simulink library "syl_grc"  (R2024a)
settings: Solver=VariableStepAuto  StartTime=0.0  StopTime=10.0  RelTol=1e-3
undefined symbols (not defined in the file or in its folder): ASYL_TrqMax_X_V, ASYL_TrqMax_Y_rpm, ASYL_TrqMin_X_V, ASYL_TrqMin_Y_rpm, KSYL_frqSwitchMax_Hz, KSYL_nTMSpdMax_RPM, KSYL_nTMSpdMin_RPM, MINUSONE_FLOAT, MSYL_TrqMax_Z_Nm, MSYL_TrqMin_Z_Nm
libraries: simulink x3
settings Model: Creator=FVT24180  LastModifiedBy=FVT22063

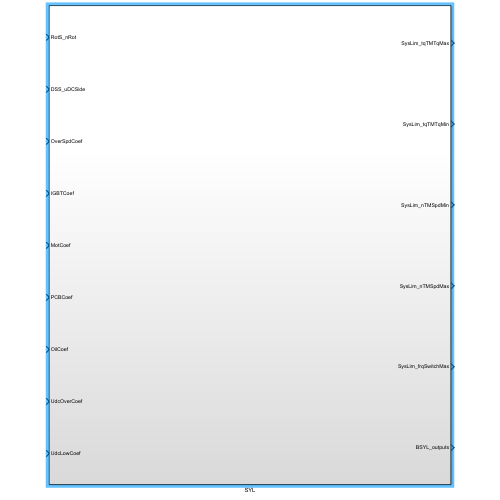
[thumbnail: Simulink's stored preview of the top-level diagram]
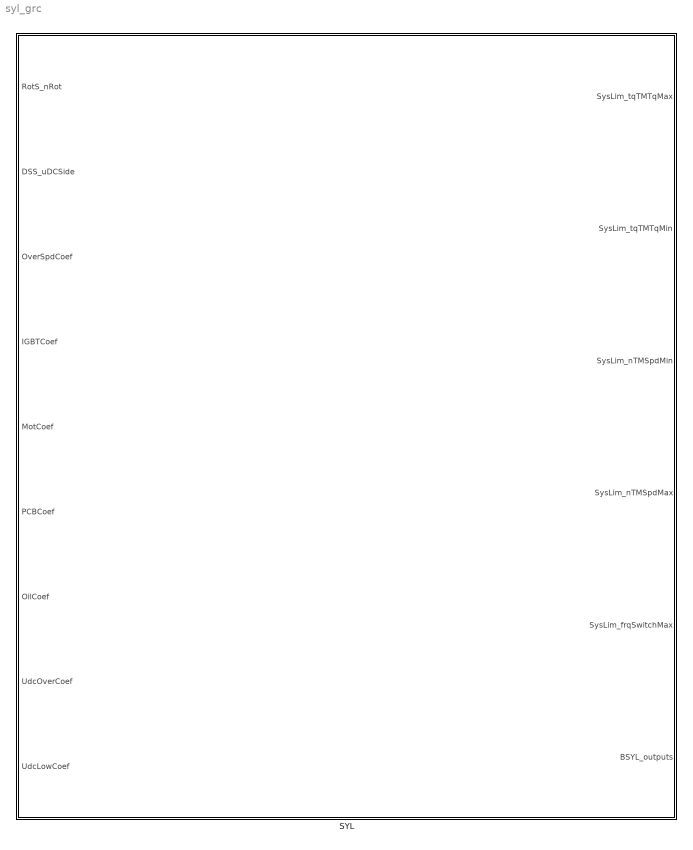
== system syl_grc ==
  SYL : Subsystem

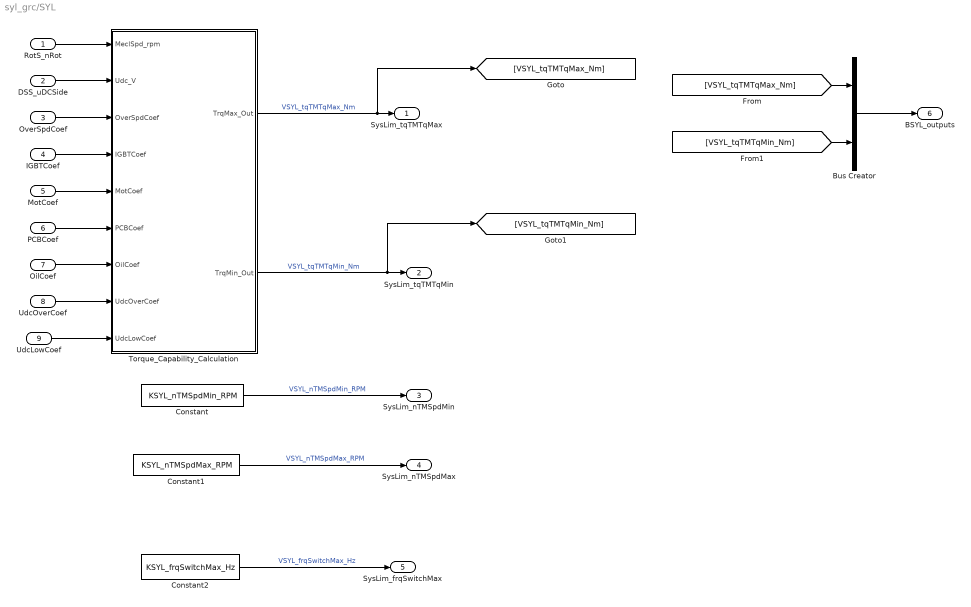
== system syl_grc/SYL ==
  RotS_nRot : Inport  OutDataTypeStr=single
  DSS_uDCSide : Inport  Port=2  OutDataTypeStr=single
  OverSpdCoef : Inport  Port=3  OutDataTypeStr=single
  IGBTCoef : Inport  Port=4  OutDataTypeStr=single
  MotCoef : Inport  Port=5  OutDataTypeStr=single
  PCBCoef : Inport  Port=6  OutDataTypeStr=single
  OilCoef : Inport  Port=7  OutDataTypeStr=single
  UdcOverCoef : Inport  Port=8  OutDataTypeStr=single
  UdcLowCoef : Inport  Port=9  OutDataTypeStr=single
  Bus Creator : BusCreator  Inputs=2  OutDataTypeStr=Bus: BSYL_outputs  NonVirtualBus=on
  Constant : Constant  Value=KSYL_nTMSpdMin_RPM  OutDataTypeStr=single
  Constant1 : Constant  Value=KSYL_nTMSpdMax_RPM  OutDataTypeStr=single
  Constant2 : Constant  Value=KSYL_frqSwitchMax_Hz  OutDataTypeStr=single
  Torque_Capability_Calculation : Subsystem  RTWFcnName=Torque_Capability_Calculation
      settings: RTWFcnNameOpts=User specified
  SysLim_tqTMTqMax : Outport  OutDataTypeStr=single  VectorParamsAs1DForOutWhenUnconnected=off
  SysLim_tqTMTqMin : Outport  Port=2  OutDataTypeStr=single  VectorParamsAs1DForOutWhenUnconnected=off
  SysLim_nTMSpdMin : Outport  Port=3  OutDataTypeStr=single  VectorParamsAs1DForOutWhenUnconnected=off
  SysLim_nTMSpdMax : Outport  Port=4  OutDataTypeStr=single  VectorParamsAs1DForOutWhenUnconnected=off
  SysLim_frqSwitchMax : Outport  Port=5  OutDataTypeStr=single  VectorParamsAs1DForOutWhenUnconnected=off
  BSYL_outputs : Outport  Port=6  OutDataTypeStr=Bus: BSYL_outputs
  wires:
  OverSpdCoef/1 -> Torque_Capability_Calculation/3(OverSpdCoef)
  UdcOverCoef/1 -> Torque_Capability_Calculation/8(UdcOverCoef)
  IGBTCoef/1 -> Torque_Capability_Calculation/4(IGBTCoef)
  Torque_Capability_Calculation/1(TrqMax_Out) -> [VSYL_tqTMTqMax_Nm], SysLim_tqTMTqMax/1  "VSYL_tqTMTqMax_Nm"
  Torque_Capability_Calculation/2(TrqMin_Out) -> [VSYL_tqTMTqMin_Nm], SysLim_tqTMTqMin/1  "VSYL_tqTMTqMin_Nm"
  RotS_nRot/1 -> Torque_Capability_Calculation/1(MeclSpd_rpm)
  PCBCoef/1 -> Torque_Capability_Calculation/6(PCBCoef)
  DSS_uDCSide/1 -> Torque_Capability_Calculation/2(Udc_V)
  Constant1/1 -> SysLim_nTMSpdMax/1  "VSYL_nTMSpdMax_RPM"
  OilCoef/1 -> Torque_Capability_Calculation/7(OilCoef)
  Constant/1 -> SysLim_nTMSpdMin/1  "VSYL_nTMSpdMin_RPM"
  MotCoef/1 -> Torque_Capability_Calculation/5(MotCoef)
  Constant2/1 -> SysLim_frqSwitchMax/1  "VSYL_frqSwitchMax_Hz"
  UdcLowCoef/1 -> Torque_Capability_Calculation/9(UdcLowCoef)
  [VSYL_tqTMTqMax_Nm] -> Bus Creator/1
  [VSYL_tqTMTqMin_Nm] -> Bus Creator/2
  Bus Creator/1 -> BSYL_outputs/1

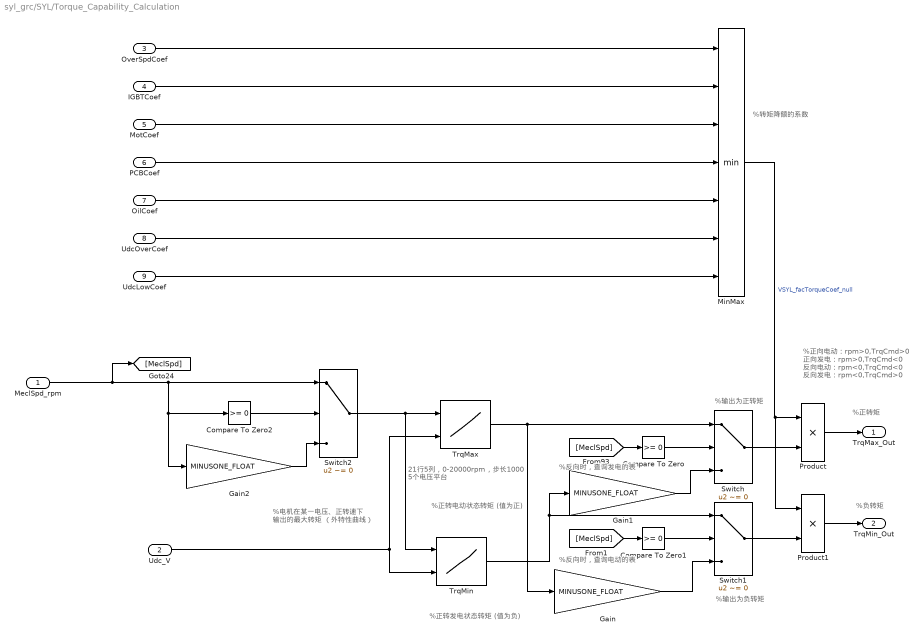
== system syl_grc/SYL/Torque_Capability_Calculation ==
  note: 21行5列，0-20000rpm，步长1000
      | 5个电压平台
  note: %负转矩
  note: %正转矩
  note: %输出为负转矩
  note: %输出为正转矩
  note: %反向时，查询电动的表
  note: %反向时，查询发电的表
  note: %正向电动：rpm>0,TrqCmd>0
      |    正向发电：rpm>0,TrqCmd<0
      |    反向电动：rpm<0,TrqCmd<0
      |    反向发电：rpm<0,TrqCmd>0
  note: %正转发电状态转矩
      | (值为负)
  note: %正转电动状态转矩
      | (值为正)
  note: %转矩降额的系数
  note: %电机在某一电压、正转速下
      | 输出的最大转矩
      | （外特性曲线）
  MeclSpd_rpm : Inport
  Udc_V : Inport  Port=2
  OverSpdCoef : Inport  Port=3  OutDataTypeStr=single
  IGBTCoef : Inport  Port=4  OutDataTypeStr=single
  MotCoef : Inport  Port=5  OutDataTypeStr=single
  PCBCoef : Inport  Port=6  OutDataTypeStr=single
  OilCoef : Inport  Port=7  OutDataTypeStr=single
  UdcOverCoef : Inport  Port=8  OutDataTypeStr=single
  UdcLowCoef : Inport  Port=9  OutDataTypeStr=single
  Compare To Zero : simulink/Logic and Bit Operations/Compare To Zero  relop=>=  OutDataTypeStr=boolean
  Compare To Zero1 : simulink/Logic and Bit Operations/Compare To Zero  relop=>=  OutDataTypeStr=boolean
  Compare To Zero2 : simulink/Logic and Bit Operations/Compare To Zero  relop=>=  OutDataTypeStr=boolean
  Gain : Gain  Gain=MINUSONE_FLOAT  OutDataTypeStr=single
  Gain1 : Gain  Gain=MINUSONE_FLOAT  OutDataTypeStr=single
  Gain2 : Gain  Gain=MINUSONE_FLOAT  OutDataTypeStr=single
  MinMax : MinMax  Inputs=7
  Product : Product
  Product1 : Product
  Switch : Switch  Criteria=u2 ~= 0  SaturateOnIntegerOverflow=off  InputSameDT=off
  Switch1 : Switch  Criteria=u2 ~= 0  SaturateOnIntegerOverflow=off  InputSameDT=off
  Switch2 : Switch  Criteria=u2 ~= 0  SaturateOnIntegerOverflow=off  InputSameDT=off
  TrqMax : Lookup_n-D  BreakpointsForDimension1=ASYL_TrqMax_Y_rpm  BreakpointsForDimension2=ASYL_TrqMax_X_V  Table=MSYL_TrqMax_Z_Nm  InternalRulePriority=Speed  RndMeth=Simplest
      settings: InputPortMap=u0,u1
  TrqMin : Lookup_n-D  BreakpointsForDimension1=ASYL_TrqMin_Y_rpm  BreakpointsForDimension2=ASYL_TrqMin_X_V  Table=MSYL_TrqMin_Z_Nm  InternalRulePriority=Speed  RndMeth=Simplest
      settings: InputPortMap=u0,u1
  TrqMax_Out : Outport  VectorParamsAs1DForOutWhenUnconnected=off
  TrqMin_Out : Outport  Port=2  VectorParamsAs1DForOutWhenUnconnected=off
  wires:
  Udc_V/1 -> TrqMax/2, TrqMin/2
  Switch2/1 -> TrqMin/1, TrqMax/1
  [MeclSpd] -> Compare To Zero/1
  Compare To Zero/1 -> Switch/2
  [MeclSpd] -> Compare To Zero1/1
  Compare To Zero1/1 -> Switch1/2
  TrqMax/1 -> Switch/1, Gain/1
  TrqMin/1 -> Gain1/1, Switch1/1
  Gain1/1 -> Switch/3
  Gain/1 -> Switch1/3
  Switch/1 -> Product/2
  Switch1/1 -> Product1/2
  MinMax/1 -> Product1/1, Product/1  "VSYL_facTorqueCoef_null"
  Product/1 -> TrqMax_Out/1
  Product1/1 -> TrqMin_Out/1
  OverSpdCoef/1 -> MinMax/1
  IGBTCoef/1 -> MinMax/2
  MotCoef/1 -> MinMax/3
  PCBCoef/1 -> MinMax/4
  OilCoef/1 -> MinMax/5
  UdcOverCoef/1 -> MinMax/6
  UdcLowCoef/1 -> MinMax/7
  Compare To Zero2/1 -> Switch2/2
  MeclSpd_rpm/1 -> Switch2/1, Compare To Zero2/1, Gain2/1, [MeclSpd]
  Gain2/1 -> Switch2/3
